simulink model "einh_puls_1"  (Simulink 7.7)
settings: Solver=ode45  StartTime=0.0  StopTime=0.01  MaxStep=1e-6  RelTol=1e-3
values from neighbouring files (symbols this model uses):
  a = zeros(5, nord+1)    [analog_tp1.m]    (also in analog_tp2.m)
  b = fir1(nr-1,0.5)    [adapt_filter1.m]    (also in adapt_filter2.m; analog_tp1.m = zeros(5, nord+1); analog_tp2.m = zeros(5, nord+1))
  dt = 1e-6    (= 1e-06)    [analog_hp12.m]    (also in analog_tp13.m = 1e-05; analog_tp2.m = 1/(10*fmin))
  k1 = 0    [analog_bp3.m]
  k2 = 1    [analog_bp3.m]
  Typ = 2    [analog_bp1.m]    (also in analog_bp2.m = 4; analog_bp3.m; analog_tp13.m; analog_tp2.m)
settings Model: Creator=svenhoffmann  LastModifiedBy=josef  ExtModeAutoUpdateStatusClock=off
settings DataIOCC: LimitDataPoints=off  MaxDataPoints=2000  SignalLoggingName=sigsOut
settings DebuggingCC: SaveWithParameterizedLinksMsg=none  SignalResolutionControl=TryResolveAllWithWarning  SolverPrmCheckMsg=none  MultiTaskDSMMsg=warning  MultiTaskCondExecSysMsg=none  StrictBusMsg=None
settings HardwareCC: TargetUnknown=on
settings RTWCC: IncludeERTFirstTime=on

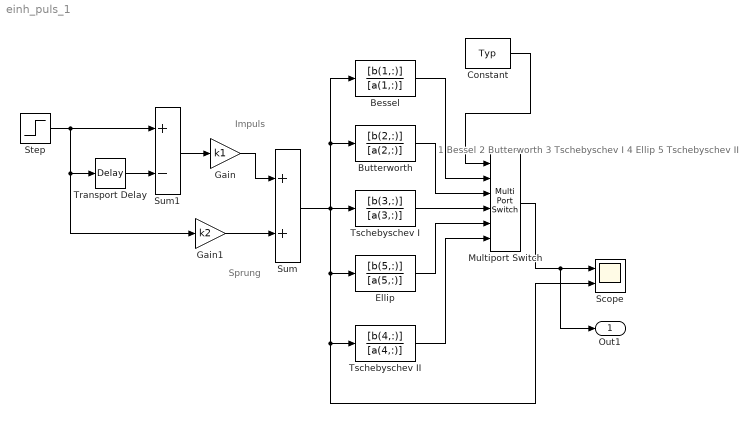
== system einh_puls_1 ==
  note: 1 Bessel
      | 2 Butterworth
      | 3 Tschebyschev I
      | 4 Ellip
      | 5 Tschebyschev II
  note: Impuls
  note: Sprung
  Bessel : TransferFcn  Numerator=[b(1,:)]  Denominator=[a(1,:)]
  Butterworth : TransferFcn  Numerator=[b(2,:)]  Denominator=[a(2,:)]
  Constant : Constant  Value=Typ
  Ellip : TransferFcn  Numerator=[b(5,:)]  Denominator=[a(5,:)]
  Gain : Gain  Gain=k1  SaturateOnIntegerOverflow=on  OutDataTypeStr=Inherit: Same as input  ParamDataTypeStr=Inherit: Same as input
  Gain1 : Gain  Gain=k2  SaturateOnIntegerOverflow=on  OutDataTypeStr=Inherit: Same as input  ParamDataTypeStr=Inherit: Same as input
  Multiport Switch : MultiPortSwitch  Inputs=5  zeroidx=off  InputSameDT=on
  Scope : Scope  NumInputPorts=2
      settings: YMin=-1~-5  YMax=1~5
  Step : Step  Time=0  SampleTime=0
  Sum : Sum  SaturateOnIntegerOverflow=on  InputSameDT=on  OutDataTypeStr=Inherit: Same as first input
  Sum1 : Sum  Inputs=+-  SaturateOnIntegerOverflow=on  InputSameDT=on  OutDataTypeStr=Inherit: Same as first input
  Transport Delay : TransportDelay  DelayTime=dt
  Tschebyschev I : TransferFcn  Numerator=[b(3,:)]  Denominator=[a(3,:)]
  Tschebyschev II : TransferFcn  Numerator=[b(4,:)]  Denominator=[a(4,:)]
  Out1 : Outport
  wires:
  Sum/1 -> Butterworth/1, Bessel/1, Tschebyschev I/1, Tschebyschev II/1, Scope/2, Ellip/1
  Bessel/1 -> Multiport Switch/2
  Butterworth/1 -> Multiport Switch/3
  Tschebyschev I/1 -> Multiport Switch/4
  Ellip/1 -> Multiport Switch/5
  Tschebyschev II/1 -> Multiport Switch/6
  Constant/1 -> Multiport Switch/1
  Multiport Switch/1 -> Scope/1, Out1/1
  Gain/1 -> Sum/1
  Gain1/1 -> Sum/2
  Step/1 -> Sum1/1, Transport Delay/1, Gain1/1
  Transport Delay/1 -> Sum1/2
  Sum1/1 -> Gain/1
